simulink model "PIcontrol"  (R2015b)
settings: Solver=FixedStepAuto  StartTime=0.0  StopTime=30  FixedStep=0.01  MaxStep=0.005  RelTol=1e-3
InitFcn:
  | Ts=0.01;
values from neighbouring files (symbols this model uses):
  A = [-1/Tg1     0      -1/(R1*Tg1)   0       0       0        0 ... (first row only)    [ObserverModel_2area.m]
  B = [ 1/Tg1 0    0    0 ... (first row only)    [ObserverModel_2area.m]
  C = [0 0 B1  1 0 0 0 ... (first row only)    [ObserverModel_2area.m]
  dPL1 = 0.    (= 0)    [ObserverModel_2area.m]
  dPL2 = 0.1    [ObserverModel_2area.m]
libraries: simulink x2
settings Model: Creator=Majidi  LastModifiedBy=Admin
settings DataIOCC: SaveFormat=Array
settings OptimizationCC: ExpressionDepthLimit=2147483647
settings DebuggingCC: UnderspecifiedInitializationDetection=Classic  MergeDetectMultiDrivingBlocksExec=none  SolverPrmCheckMsg=warning  StateNameClashWarn=warning
settings HardwareCC: ProdBitPerPointer=32  ProdLargestAtomicFloat=None  ProdIntDivRoundTo=Undefined  ProdEndianess=Unspecified  ProdWordSize=32  ProdHWDeviceType=32-bit Generic
settings GRTTargetCC: GeneratePreprocessorConditionals=Disable all
settings ConfigComp: CovModelRefEnable=Off

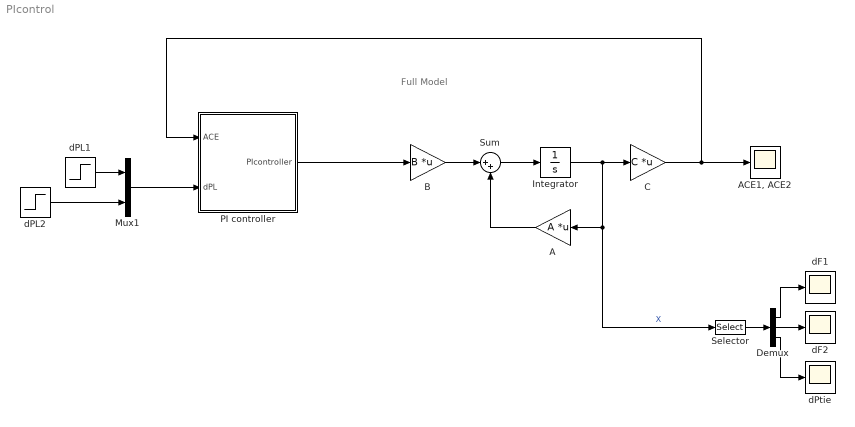
== system PIcontrol ==
  note: Full Model
  A : Gain  Gain=A  Multiplication=Matrix(K*u)
  "ACE1, ACE2" : Scope
  B : Gain  Gain=B  Multiplication=Matrix(K*u)
  C : Gain  Gain=C  Multiplication=Matrix(K*u)
  Demux : Demux  Outputs=3
  Integrator : Integrator
  Mux1 : Mux  Inputs=2
  PI controller : Subsystem
  Selector : Selector  InputPortWidth=7  IndexOptions=Index vector (dialog)  Indices=[3 7 4]  OutputSizes=1
  Sum : Sum  Inputs=|++
  dF1 : Scope
  dF2 : Scope
  dPL1 : Step  After=dPL1  SampleTime=0
  dPL2 : Step  After=dPL2  SampleTime=0
  dPtie : Scope
  wires:
  B/1 -> Sum/1
  Sum/1 -> Integrator/1
  A/1 -> Sum/2
  Integrator/1 -> A/1, Selector/1, C/1  "X"
  C/1 -> PI controller/1(ACE), "ACE1, ACE2"/1
  dPL1/1 -> Mux1/1
  dPL2/1 -> Mux1/2
  Demux/1 -> dF1/1
  Demux/2 -> dF2/1
  Demux/3 -> dPtie/1
  Selector/1 -> Demux/1
  Mux1/1 -> PI controller/2(dPL)
  PI controller/1(PIcontroller) -> B/1

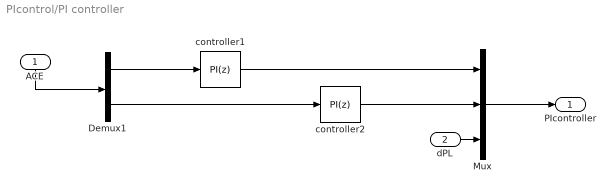
== system PIcontrol/PI controller ==
  ACE : Inport
  dPL : Inport  Port=2
  Demux1 : Demux  Outputs=2
  Mux : Mux  Inputs=3
  controller1 : simulink/Continuous/PID Controller  Controller=PI  TimeDomain=Discrete-time  SampleTime=-1  IntegratorMethod=Forward Euler  FilterMethod=Forward Euler  Form=Parallel  UseFilter=on  ControllerParametersSource=internal  P=0.2424  I=-0.3620  D=0  N=100  InitialConditionSource=internal  InitialConditionForIntegrator=0  InitialConditionForFilter=0  ExternalReset=none  LimitOutput=off  UpperSaturationLimit=0.25  LowerSaturationLimit=-0.25  LinearizeAsGain=off  AntiWindupMode=none  Kb=1  TrackingMode=off  Kt=1  PParamMin=[]  PParamMax=[]  IParamMin=[]  IParamMax=[]  DParamMin=[]  DParamMax=[]  NParamMin=[]  NParamMax=[]  KbParamMin=[]  KbParamMax=[]  KtParamMin=[]  KtParamMax=[]  POutMin=[]  POutMax=[]  IOutMin=[]  IOutMax=[]  DOutMin=[]  DOutMax=[]  NOutMin=[]  NOutMax=[]  KbOutMin=[]  KbOutMax=[]  KtOutMin=[]  KtOutMax=[]  IntegratorOutMin=[]  IntegratorOutMax=[]  FilterOutMin=[]  FilterOutMax=[]  SumOutMin=[]  SumOutMax=[]  SumI1OutMin=[]  SumI1OutMax=[]  SumI2OutMin=[]  SumI2OutMax=[]  SumI3OutMin=[]  SumI3OutMax=[]  SumDOutMin=[]  SumDOutMax=[]  SaturationOutMin=[]  SaturationOutMax=[]  IntegratorContinuousStateAttributes=''  IntegratorStateMustResolveToSignalObject=off  IntegratorRTWStateStorageClass=Auto  FilterContinuousStateAttributes=''  FilterStateMustResolveToSignalObject=off  FilterRTWStateStorageClass=Auto  DifferentiatorICPrevScaledInput=0  DifferentiatorOutMin=[]  DifferentiatorOutMax=[]
  controller2 : simulink/Continuous/PID Controller  Controller=PI  TimeDomain=Discrete-time  SampleTime=-1  IntegratorMethod=Forward Euler  FilterMethod=Forward Euler  Form=Parallel  UseFilter=on  ControllerParametersSource=internal  P=0.1821  I=-0.3713  D=0  N=100  InitialConditionSource=internal  InitialConditionForIntegrator=0  InitialConditionForFilter=0  ExternalReset=none  LimitOutput=off  UpperSaturationLimit=0.25  LowerSaturationLimit=-0.25  LinearizeAsGain=off  AntiWindupMode=none  Kb=1  TrackingMode=off  Kt=1  PParamMin=[]  PParamMax=[]  IParamMin=[]  IParamMax=[]  DParamMin=[]  DParamMax=[]  NParamMin=[]  NParamMax=[]  KbParamMin=[]  KbParamMax=[]  KtParamMin=[]  KtParamMax=[]  POutMin=[]  POutMax=[]  IOutMin=[]  IOutMax=[]  DOutMin=[]  DOutMax=[]  NOutMin=[]  NOutMax=[]  KbOutMin=[]  KbOutMax=[]  KtOutMin=[]  KtOutMax=[]  IntegratorOutMin=[]  IntegratorOutMax=[]  FilterOutMin=[]  FilterOutMax=[]  SumOutMin=[]  SumOutMax=[]  SumI1OutMin=[]  SumI1OutMax=[]  SumI2OutMin=[]  SumI2OutMax=[]  SumI3OutMin=[]  SumI3OutMax=[]  SumDOutMin=[]  SumDOutMax=[]  SaturationOutMin=[]  SaturationOutMax=[]  IntegratorContinuousStateAttributes=''  IntegratorStateMustResolveToSignalObject=off  IntegratorRTWStateStorageClass=Auto  FilterContinuousStateAttributes=''  FilterStateMustResolveToSignalObject=off  FilterRTWStateStorageClass=Auto  DifferentiatorICPrevScaledInput=0  DifferentiatorOutMin=[]  DifferentiatorOutMax=[]
  PIcontroller : Outport
  wires:
  Demux1/1 -> controller1/1
  ACE/1 -> Demux1/1
  dPL/1 -> Mux/3
  Mux/1 -> PIcontroller/1
  Demux1/2 -> controller2/1
  controller1/1 -> Mux/1
  controller2/1 -> Mux/2
